simulink model "Example_1"  (R2017b)
settings: Solver=VariableStepAuto  StartTime=0.0  StopTime=T_stop  MaxStep=Max_step  MinStep=Min_step  RelTol=1e-3
values from neighbouring files (symbols this model uses):
  C1 = 4E-6    (= 4e-06)    [Example_01.m]
  L1 = (G*C_SS)    [AC_L15_Example1.m]    (also in AC_L15_Example2.m = C_SS*G; AC_L16_1.m = G*C_SS; AC_L16_2.m = C_SS*G; AC_L17.m = G*C_SS)
  R1 = 68    [Example_01.m]
  x0 = [0;0]    [Example_01.m]
settings Model: Creator=hantao.li  LastModifiedBy=hantao.li

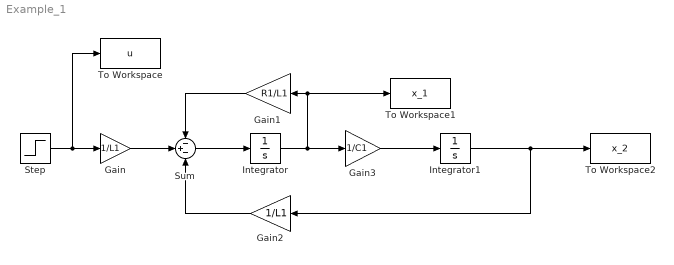
== system Example_1 ==
  Gain : Gain  Gain=1/L1
  Gain1 : Gain  Gain=R1/L1
  Gain2 : Gain  Gain=1/L1
  Gain3 : Gain  Gain=1/C1
  Integrator : Integrator  InitialCondition=x0(1)
  Integrator1 : Integrator  InitialCondition=x0(2)
  Step : Step  Time=0  SampleTime=0
  Sum : Sum  Inputs=-+-
  To Workspace : ToWorkspace  VariableName=u  SaveFormat=Timeseries  SampleTime=-1
  To Workspace1 : ToWorkspace  VariableName=x_1  SaveFormat=Timeseries  SampleTime=-1
  To Workspace2 : ToWorkspace  VariableName=x_2  SaveFormat=Timeseries  SampleTime=-1
  wires:
  Step/1 -> To Workspace/1, Gain/1
  Gain/1 -> Sum/2
  Sum/1 -> Integrator/1
  Gain1/1 -> Sum/1
  Gain2/1 -> Sum/3
  Integrator/1 -> To Workspace1/1, Gain1/1, Gain3/1
  Gain3/1 -> Integrator1/1
  Integrator1/1 -> Gain2/1, To Workspace2/1
